simulink model "FullVehicleModel_ABS_ESP"  (R2019a)
settings: Solver=ode23s  StartTime=0.0  StopTime=t_f  MaxStep=0.1  RelTol=1e-3
values from neighbouring files (symbols this model uses):
  acc_US_test = 0    [mainVehicleModel.m]
  auxiliary_data = block.DialogPrm(3).Data    [FullVehicleModel_V3_sfun.m]    (also in mainVehicleModel.m = getAuxiliaryDataStruct())
  curv_akermann = 0    [mainVehicleModel.m]
  hv = 0.5    [mainVehicleModel.m]
  init_conditions_data = getInitialConditionsDataStruct( V_init )    [mainVehicleModel.m]
  lambda1_th = 0.2    [mainVehicleModel.m]
  lambda2_th = 0.1    [mainVehicleModel.m]
  maneuver_flag = 4    [mainVehicleModel.m]
  parametri_ABS = para    [ABSParameters.m]    (also in mainVehicleModel.m = ABSParameters(getVehicleDataStruct()))
  rho_off = 0.9    [mainVehicleModel.m]
  rho_on = 1.02    [mainVehicleModel.m]
  t_brake = t_f+1    (= 61)    [mainVehicleModel.m]
  Tb_dot_max = 5000    [mainVehicleModel.m]
  V_init = 50    [mainVehicleModel.m]
  v_on = 2.5    [mainVehicleModel.m]
  v_stop = 0.1    [mainVehicleModel.m]
  vehicle_data = block.DialogPrm(1).Data    [FullVehicleModel_V3_sfun.m]    (also in mainVehicleModel.m = getVehicleDataStruct())
undefined symbols (not defined in the file or in its folder): magnitude, sigbuilder_block
libraries: simulink x6, dspsigops x4
(part 1 of 2)
settings Model: Creator=luca  LastModifiedBy=LorenzoZappata
settings DataIOCC: SaveFormat=Array  ReturnWorkspaceOutputs=off
settings DebuggingCC: ArithmeticOperatorsInVariantConditions=warning
settings SFSimCC: SimUseLocalCustomCode=off
settings RTWCC: RTWUseLocalCustomCode=off
settings CodeAppCC: StateflowObjectComments=on

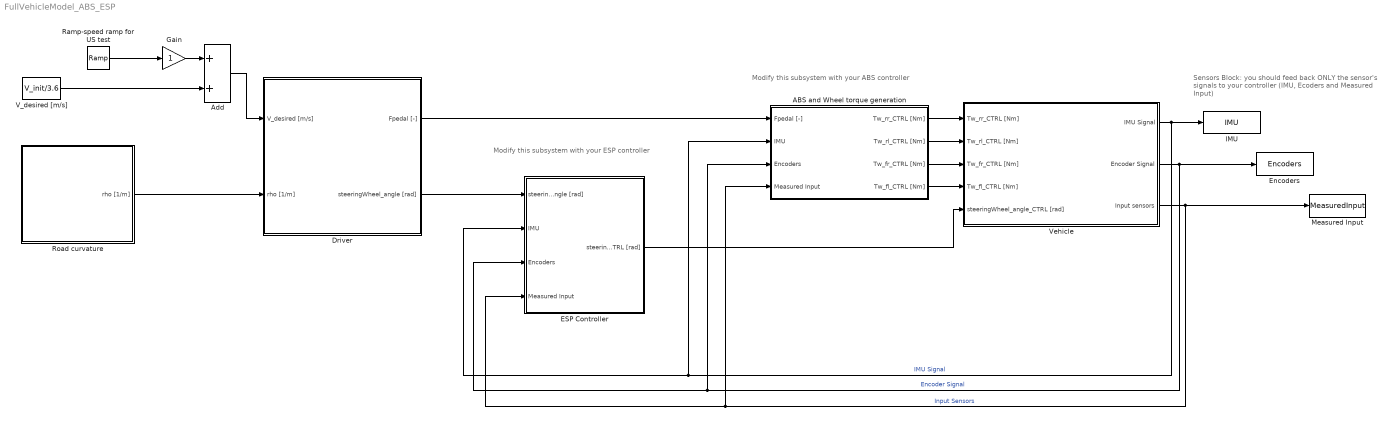
== system FullVehicleModel_ABS_ESP ==
  note: Modify this subsystem with your ABS controller
  note: Modify this subsystem with your ESP
      | controller
  note: Sensors Block: you should feed back ONLY
      | the sensor's signals to your controller
      | (IMU, Ecoders and Measured Input)
  ABS and Wheel torque generation : Subsystem
  Add : Sum
  Driver : Subsystem
  ESP Controller : Subsystem
  Encoders : ToWorkspace  VariableName=Encoders  SaveFormat=Timeseries  SampleTime=-1
  Gain : Gain
  IMU : ToWorkspace  VariableName=IMU  SaveFormat=Timeseries  SampleTime=-1
  Measured Input : ToWorkspace  VariableName=MeasuredInput  SaveFormat=Timeseries  SampleTime=-1
  Ramp-speed ramp for US test : simulink/Sources/Ramp  slope=acc_US_test  start=Tstart_US_test  InitialOutput=0
  Road curvature : Subsystem
  V_desired [m/s] : Constant  Value=V_init/3.6
  Vehicle : Subsystem
  wires:
  Driver/1(Fpedal [-]) -> ABS and Wheel torque generation/1(Fpedal [-])
  Driver/2(steeringWheel_angle [rad]) -> ESP Controller/1(steeringWheel_angle [rad])
  Vehicle/1(IMU Signal) -> IMU/1, ABS and Wheel torque generation/2(IMU), ESP Controller/2(IMU)  "IMU Signal"
  Vehicle/2(Encoder Signal) -> Encoders/1, ABS and Wheel torque generation/3(Encoders), ESP Controller/3(Encoders)  "Encoder Signal"
  Vehicle/3(Input sensors) -> Measured Input/1, ABS and Wheel torque generation/4(Measured Input), ESP Controller/4(Measured Input)  "Input Sensors"
  ESP Controller/1(steeringWheel_angle_CTRL [rad]) -> Vehicle/5(steeringWheel_angle_CTRL [rad])
  ABS and Wheel torque generation/4(Tw_fl_CTRL [Nm]) -> Vehicle/4(Tw_fl_CTRL [Nm])
  ABS and Wheel torque generation/3(Tw_fr_CTRL [Nm]) -> Vehicle/3(Tw_fr_CTRL [Nm])
  ABS and Wheel torque generation/2(Tw_rl_CTRL [Nm]) -> Vehicle/2(Tw_rl_CTRL [Nm])
  ABS and Wheel torque generation/1(Tw_rr_CTRL [Nm]) -> Vehicle/1(Tw_rr_CTRL [Nm])
  Ramp-speed ramp for US test/1 -> Gain/1
  V_desired [m/s]/1 -> Add/2
  Add/1 -> Driver/1(V_desired [m/s])
  Gain/1 -> Add/1
  Road curvature/1(rho [1/m]) -> Driver/2(rho [1/m])

== system FullVehicleModel_ABS_ESP/ABS and Wheel torque generation ==
  note: Insert your ABS design in the
      | following Subsystems
  Fpedal [-] : Inport
  IMU : Inport  Port=2
  Encoders : Inport  Port=3
  Measured Input : Inport  Port=4
  ABS Front Left Wheel : Subsystem
  ABS Front Right Wheel : Subsystem
  ABS Rear Left Wheel : Subsystem
  ABS Rear Right Wheel : Subsystem
  Accelerator : Subsystem
  Brake : Subsystem
  Demux : Demux
  Scope6 : Scope
  Switch : Switch
  Tw_rr_CTRL [Nm] : Outport
  Tw_rl_CTRL [Nm] : Outport  Port=2
  Tw_fr_CTRL [Nm] : Outport  Port=3
  Tw_fl_CTRL [Nm] : Outport  Port=4
  wires:
  Demux/2 -> ABS Rear Left Wheel/1(Tw_rl [Nm])
  Switch/1 -> Demux/1
  Demux/1 -> Scope6/1, ABS Rear Right Wheel/1(Tw_rr [Nm])
  Fpedal [-]/1 -> Brake/1(Fpedal [-]), Accelerator/1(Fpedal [-]), Switch/2
  ABS Rear Right Wheel/1(Tw_rr_CTRL [Nm]) -> Tw_rr_CTRL [Nm]/1
  Measured Input/1 -> ABS Front Left Wheel/4(Measured Input), ABS Front Right Wheel/4(Measured Input), ABS Rear Left Wheel/4(Measured Input), ABS Rear Right Wheel/4(Measured Input)
  Encoders/1 -> ABS Rear Right Wheel/3(Encoders), ABS Front Right Wheel/3(Encoders), ABS Front Left Wheel/3(Encoders), ABS Rear Left Wheel/3(Encoders)
  IMU/1 -> ABS Rear Left Wheel/2(IMU), ABS Front Left Wheel/2(IMU), ABS Front Right Wheel/2(IMU), ABS Rear Right Wheel/2(IMU)
  ABS Rear Left Wheel/1(Tw_rl_CTRL [Nm]) -> Tw_rl_CTRL [Nm]/1
  Demux/3 -> ABS Front Right Wheel/1(Tw_fr [Nm])
  ABS Front Right Wheel/1(Tw_rr_CTRL [Nm]) -> Tw_fr_CTRL [Nm]/1
  Demux/4 -> ABS Front Left Wheel/1(Tw_fl [Nm])
  ABS Front Left Wheel/1(Tw_rr_CTRL [Nm]) -> Tw_fl_CTRL [Nm]/1
  Accelerator/1(Tw [Nm]) -> Switch/1
  Brake/1(Tw [Nm]) -> Switch/3

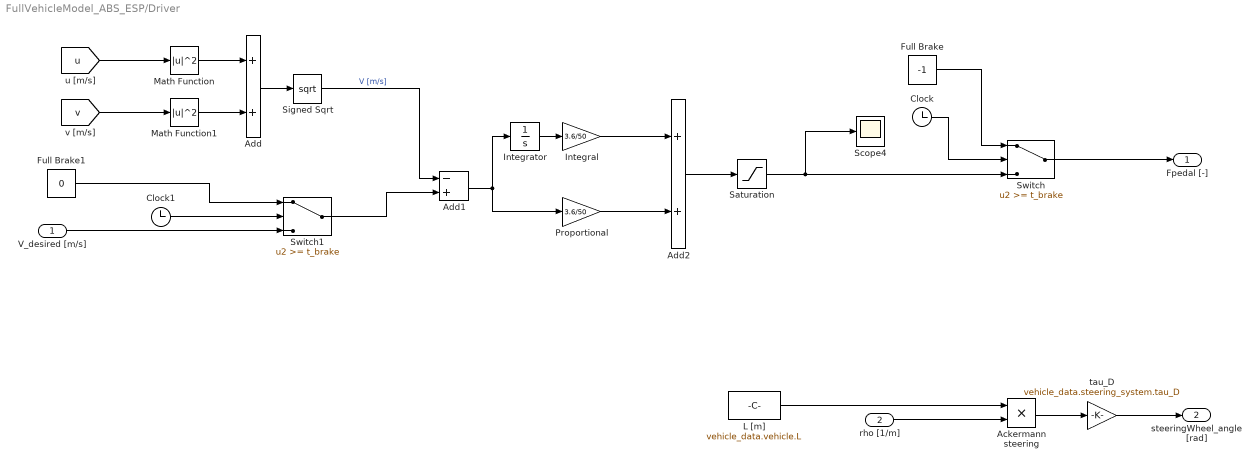
== system FullVehicleModel_ABS_ESP/Driver ==
  V_desired [m/s] : Inport
  rho [1/m] : Inport  Port=2
  Ackermann steering : Product  Inputs=**
  Add : Sum
  Add1 : Sum  Inputs=-+
  Add2 : Sum
  Clock : Clock
  Clock1 : Clock
  Full Brake : Constant  Value=-1
  Full Brake1 : Constant  Value=0
  Integral : Gain  Gain=3.6/50
  Integrator : Integrator
  L [m] : Constant  Value=vehicle_data.vehicle.L
  Math Function : Math  Operator=magnitude^2  SaturateOnIntegerOverflow=on
  Math Function1 : Math  Operator=magnitude^2  SaturateOnIntegerOverflow=on
  Proportional : Gain  Gain=3.6/50
  Saturation : Saturate  UpperLimit=1  LowerLimit=-1
  Scope4 : Scope
  Signed Sqrt : Sqrt  SaturateOnIntegerOverflow=on
  Switch : Switch  Threshold=t_brake
  Switch1 : Switch  Threshold=t_brake
  tau_D : Gain  Gain=vehicle_data.steering_system.tau_D
  Fpedal [-] : Outport
  steeringWheel_angle [rad] : Outport  Port=2
  wires:
  Proportional/1 -> Add2/2
  Add2/1 -> Saturation/1
  Integrator/1 -> Integral/1
  L [m]/1 -> Ackermann steering/1
  Add/1 -> Signed Sqrt/1
  Math Function1/1 -> Add/2
  Add1/1 -> Integrator/1, Proportional/1
  Signed Sqrt/1 -> Add1/1  "V [m/s]"
  Ackermann steering/1 -> tau_D/1
  Math Function/1 -> Add/1
  rho [1/m]/1 -> Ackermann steering/2
  Integral/1 -> Add2/1
  [u] -> Math Function/1
  [v] -> Math Function1/1
  V_desired [m/s]/1 -> Switch1/3
  Saturation/1 -> Switch/3, Scope4/1
  Full Brake1/1 -> Switch1/1
  Clock1/1 -> Switch1/2
  Full Brake/1 -> Switch/1
  Clock/1 -> Switch/2
  Switch/1 -> Fpedal [-]/1
  Switch1/1 -> Add1/2
  tau_D/1 -> steeringWheel_angle [rad]/1

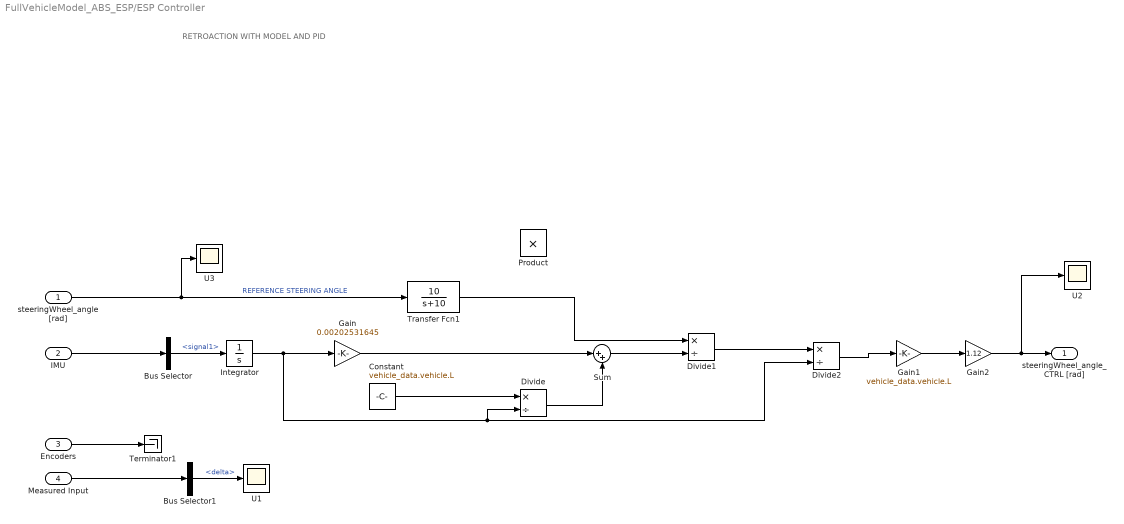
== system FullVehicleModel_ABS_ESP/ESP Controller ==
  note: RETROACTION WITH MODEL AND PID
  steeringWheel_angle [rad] : Inport
  IMU : Inport  Port=2
  Encoders : Inport  Port=3
  Measured Input : Inport  Port=4
  Bus Selector : BusSelector  OutputSignals=signal1
  Bus Selector1 : BusSelector  OutputSignals=delta
  Constant : Constant  Value=vehicle_data.vehicle.L
  Divide : Product  Inputs=*/
  Divide1 : Product  Inputs=*/
  Divide2 : Product  Inputs=*/
  Gain : Gain  Gain=0.00202531645
  Gain1 : Gain  Gain=vehicle_data.vehicle.L
  Gain2 : Gain  Gain=1.12
  Integrator : Integrator  InitialCondition=V_init/3.6
  Product : Product
  Sum : Sum  Inputs=|++
  Terminator1 : Terminator
  Transfer Fcn1 : TransferFcn  Numerator=[10]  Denominator=[1 10]
  U1 : Scope
  U2 : Scope
  U3 : Scope
  steeringWheel_angle_CTRL [rad] : Outport
  wires:
  Encoders/1 -> Terminator1/1
  Measured Input/1 -> Bus Selector1/1
  Integrator/1 -> Gain/1, Divide2/2, Divide/2
  IMU/1 -> Bus Selector/1
  Bus Selector/1 -> Integrator/1  "<signal1>"
  steeringWheel_angle [rad]/1 -> Transfer Fcn1/1, U3/1  "REFERENCE STEERING ANGLE"
  Constant/1 -> Divide/1
  Gain/1 -> Sum/1
  Divide/1 -> Sum/2
  Sum/1 -> Divide1/2
  Divide1/1 -> Divide2/1
  Divide2/1 -> Gain1/1
  Gain2/1 -> U2/1, steeringWheel_angle_CTRL [rad]/1
  Gain1/1 -> Gain2/1
  Transfer Fcn1/1 -> Divide1/1
  Bus Selector1/1 -> U1/1  "<delta>"

== system FullVehicleModel_ABS_ESP/Road curvature ==
  1/(tau_D) : Gain  Gain=1/(vehicle_data.steering_system.tau_D)
  1/(tau_D)1 : Gain  Gain=1/(vehicle_data.steering_system.tau_D)
  1/(tau_D)2 : Gain  Gain=1/(vehicle_data.steering_system.tau_D)
  Brake Maneuver : Constant  Value=0
  Constant curvature Maneuver : Subsystem  Tag=STV Subsys  LoadFcn=sigbuilder_block('load');  StartFcn=sigbuilder_block('start');  StopFcn=sigbuilder_block('stop');  ClipboardFcn=sigbuilder_block('clipboard');  mask(Sigbuilder block){tuvar=[0:10]}
      mask help: Simulink:masks:SigbuilderBlock_MD
      mask init:
      | if ~strcmp(get_param(bdroot(gcbh),'SimulationStatus'),'stopped') tuvar = sigbuilder_block('maskInit'); end
      settings: CopyFcn=sigbuilder_block('copy');  DeleteFcn=sigbuilder_block('delete');  ModelCloseFcn=sigbuilder_block('modelClose');  PreSaveFcn=sigbuilder_block('preSave');  PauseFcn=sigbuilder_block('pause');  ContinueFcn=sigbuilder_block('continue');  NameChangeFcn=sigbuilder_block('namechange');  OpenFcn=sigbuilder_block('open',[0 0 1319 754 ]);  CloseFcn=sigbuilder_block('close');
      mask Display: plot(0, 0, 100, 100,[2, 2, 32, 32, 2], [68, 8, 8, 68, 68],[32, 2], [38, 38], [32, 19, 2],[53, 60, 44], [32, 17, 17, 2],[16, 16, 31, 31]);txt = getActiveGroup(gcbh);text(2, 100, txt,'verticalAlignment', 'top');
  Desired curvature  [1/m] : Constant  Value=curv_akermann
  Double Lane Change Maneuver : Subsystem  Tag=STV Subsys  LoadFcn=sigbuilder_block('load');  StartFcn=sigbuilder_block('start');  StopFcn=sigbuilder_block('stop');  ClipboardFcn=sigbuilder_block('clipboard');  mask(Sigbuilder block){tuvar=[0:10]}
      mask help: Simulink:masks:SigbuilderBlock_MD
      mask init:
      | if ~strcmp(get_param(bdroot(gcbh),'SimulationStatus'),'stopped') tuvar = sigbuilder_block('maskInit'); end
      settings: CopyFcn=sigbuilder_block('copy');  DeleteFcn=sigbuilder_block('delete');  ModelCloseFcn=sigbuilder_block('modelClose');  PreSaveFcn=sigbuilder_block('preSave');  PauseFcn=sigbuilder_block('pause');  ContinueFcn=sigbuilder_block('continue');  NameChangeFcn=sigbuilder_block('namechange');  OpenFcn=sigbuilder_block('open',[0 0 1280 649 ]);  CloseFcn=sigbuilder_block('close');
      mask Display: plot(0, 0, 100, 100,[2, 2, 32, 32, 2], [68, 8, 8, 68, 68],[32, 2], [38, 38], [32, 19, 2],[53, 60, 44], [32, 17, 17, 2],[16, 16, 31, 31]);txt = getActiveGroup(gcbh);text(2, 100, txt,'verticalAlignment', 'top');
  Maneuver Flag : Constant  Value=maneuver_flag
  Multiport Switch : MultiPortSwitch  Inputs=4
  Product : Product
  Step : Step  SampleTime=0
  rho [1/m] : Outport
  wires:
  Brake Maneuver/1 -> 1/(tau_D)/1
  Maneuver Flag/1 -> Multiport Switch/1
  Constant curvature Maneuver/1(Signal 1) -> 1/(tau_D)2/1
  Double Lane Change Maneuver/1(Signal 1) -> 1/(tau_D)1/1
  Multiport Switch/1 -> rho [1/m]/1
  Desired curvature  [1/m]/1 -> Product/2
  Product/1 -> Multiport Switch/5
  Step/1 -> Product/1
  1/(tau_D)/1 -> Multiport Switch/2
  1/(tau_D)1/1 -> Multiport Switch/3
  1/(tau_D)2/1 -> Multiport Switch/4

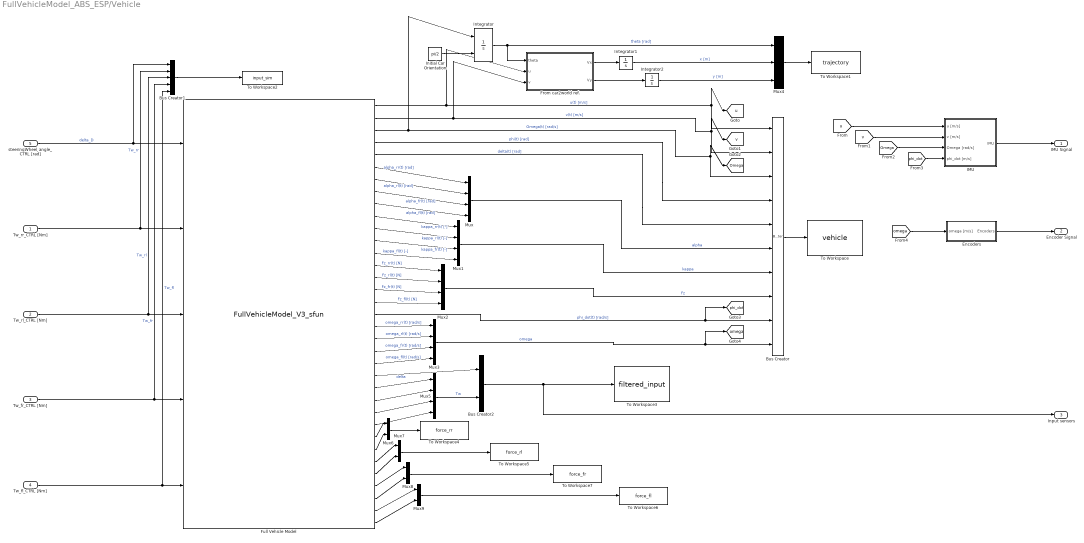
== system FullVehicleModel_ABS_ESP/Vehicle ==
  Tw_rr_CTRL [Nm] : Inport
  Tw_rl_CTRL [Nm] : Inport  Port=2
  Tw_fr_CTRL [Nm] : Inport  Port=3
  Tw_fl_CTRL [Nm] : Inport  Port=4
  steeringWheel_angle_CTRL [rad] : Inport  Port=5
  Bus Creator : BusCreator  Inputs=10
  Bus Creator1 : BusCreator  Inputs=5
  Bus Creator2 : BusCreator  Inputs=2
  Encoders : Subsystem
  "From car2world ref. " : Subsystem
  Full Vehicle Model : M-S-Function  FunctionName=FullVehicleModel_V3_sfun  Parameters=vehicle_data, init_conditions_data, auxiliary_data  mask(Matlab S-function:FullVehicleModel_V3_sfun){vehicle_data=vehicle_data, init_conditions_data=init_conditions_data, auxiliary_data=auxiliary_data}
      mask prompts: vehicle_data "Vehicle data structure"; init_conditions_data "Initial conditions structure"; auxiliary_data "Auxiliary data"
      mask help: This is a level-2 MATLAB file S-function that implements full vehicle dynamics at high and low speeds. This includes the vertical and lateral dynamics, together with wheel dynamics (wheels speed, lateral and longitudinal slip) and roll dynamics.
      mask Display:
      | port_label('input', 1, 'delta_D [rad]');
      | port_label('input', 2, 'Tw_rr [Nm]');
      | port_label('input', 3, 'Tw_rl [Nm]');
      | port_label('input', 4, 'Tw_fr [Nm]');
      | port_label('input', 5, 'Tw_fl [Nm]');
      | 
      | % x(1)  = u(t)        -> Longitudinal vehicle velocity
      | port_label('output', 1, 'u [m/s]');
      | % x(2)  = v(t)        -> Lateral vehicle velocity
      | port_label('output', 2, 'v [m/s]');
      | % x(3)  = Omega(t)    -> Yaw rate
      | port_label('output', 3, 'Omega [rad/s]');
      | % x(4)  = phi(t)      -> Roll angle
      | port_label('output', 4, 'phi [rad]');
      | % x(5)  = delta(t)    -> Steering angle
      | port_label('output', 5, 'delta [rad]');
      | % x(6)  = alpha_rr(t) -> Side slip angle, rear right wheel
      | port_label('output', 6, 'alpha_rr [-]');
      | % x(7)  = alpha_rl(t) -> Side slip angle, rear left wheel
      | port_label('output', 7, 'alpha_rl [-]');
      | % x(8)  = alpha_fr(t) -> Side slip angle, front right wheel
      | port_label('output', 8, 'alpha_fr [-]');
      | % x(9)  = alpha_fl(t) -> Side slip angle, front left wheel
      | port_label('output', 9, 'alpha_fl [-]');
      | % x(10) = kappa_rr(t) -> Longitudinal slip, rear right wheel
      | port_label('output', 10, 'kappa_rr [-]');
      | % x(11) = kappa_rl(t) -> Longitudinal slip, rear left wheel
      | port_label('output', 11, 'kappa_rl [-]');
      | % x(12) = kappa_fr(t) -> Longitudinal slip, front right wheel
      | port_label('output', 12, 'kappa_fr [-]');
      | % x(13) = kappa_fl(t) -> Longitudinal slip, front left wheel
      | port_label('output', 13, 'kappa_fl [-]');
      | % x(14) = Fz_rr(t)    -> Vertical load, rear right wheel
      | port_label('output', 14, 'Fz_rr [N]');
      | % x(15) = Fz_rl(t)    -> Vertical load, rear rear left wheel
      | port_label('output', 15, 'Fz_rl [N]');
      | % x(16) = Fz_fr(t)    -> Vertical load, front right wheel
      | port_label('output', 16, 'Fz_fr [N]');
      | % x(17) = Fz_fl(t)    -> Vertical load, front left wheel
      | port_label('output', 17, 'Fz_fl [N]');
      | % x(18) = phi_dot(t)  -> Roll rate
      | port_label('output', 18, 'phi_dot [rad/s]');
      | % x(19) = omega_rr(t) -> angular velocity rear right wheel
      | port_label('output', 19, 'omega_rr [rad/s]');
      | % x(20) = omega_rl(t) -> angular velocity rear left wheel
      | port_label('output', 20, 'omega_rl [rad/s]');
      | % x(21) = omega_fr(t) -> angular velocity front right wheel
      | port_label('output', 21, 'omega_fr [rad/s]');
      | % x(22) = omega_fl(t) -> angular velocity front left wheel
      | port_label('output', 22, 'omega_fl [rad/s]');
      | % x(23) = delta(t) -> real steer angle
      | port_label('output', 23, 'delta [rad]');
      | % x(24:27) = Tw(t) -> Filtered wheel torque
      | port_label('output', 24, 'Tw_rr [Nm]');
      | port_label('output', 25, 'Tw_rl [Nm]');
      | port_label('output', 26, 'Tw_fr [Nm]');
      | port_label('output', 27, 'Tw_fl [Nm]');
      | 
      | % Wheel forces
      | % Rear Right
      | port_label('output', 28, 'Fx_rr [N]');
      | port_label('output', 29, 'Fy_rr [N]');
      | % Rear Left
      | port_label('output', 30, 'Fx_rl [N]');
      | port_label('output', 31, 'Fy_rl [N]');
      | % Front Right
      | port_label('output', 32, 'Fx_fr [N]');
      | port_label('output', 33, 'Fy_fr [N]');
      | % Front Left
      | port_label('output', 34, 'Fx_fl [N]');
      | port_label('output', 35, 'Fy_fl [N]');
  IMU : Subsystem
  Initial Car Orientation : Constant  Value=pi/2
  Integrator : Integrator  InitialConditionSource=external
  Integrator1 : Integrator
  Integrator2 : Integrator
  Mux{,1..3,5} (5 alike) : Mux
  Mux4 : Mux  Inputs=3
  Mux{6..9} (4 alike) : Mux  Inputs=2
  To Workspace : ToWorkspace  VariableName=vehicle  SaveFormat=Timeseries  SampleTime=-1
  To Workspace1 : ToWorkspace  VariableName=trajectory  SaveFormat=Timeseries  SampleTime=-1
  To Workspace2 : ToWorkspace  VariableName=input_sim  SaveFormat=Timeseries  SampleTime=-1
  To Workspace3 : ToWorkspace  VariableName=filtered_input  SaveFormat=Timeseries  SampleTime=-1
  To Workspace4 : ToWorkspace  VariableName=force_rr  SaveFormat=Timeseries  SampleTime=-1
  To Workspace5 : ToWorkspace  VariableName=force_rl  SaveFormat=Timeseries  SampleTime=-1
  To Workspace6 : ToWorkspace  VariableName=force_fl  SaveFormat=Timeseries  SampleTime=-1
  To Workspace7 : ToWorkspace  VariableName=force_fr  SaveFormat=Timeseries  SampleTime=-1
  IMU Signal : Outport
  Encoder Signal : Outport  Port=2
  Input sensors : Outport  Port=3
  tag scope: Omega=global, omega=global, phi_dot=global, u=global, v=global
  wires:
  Mux5/1 -> Bus Creator2/2  "Tw"
  Full Vehicle Model/4 -> Bus Creator/4  "phi(t) [rad]"
  Integrator/1 -> "From car2world ref. "/1(theta), Mux4/1  "theta [rad]"
  Mux8/1 -> To Workspace7/1
  Full Vehicle Model/32 -> Mux8/1
  Mux2/1 -> Bus Creator/8  "Fz"
  "From car2world ref. "/1(Vx) -> Integrator1/1
  Full Vehicle Model/28 -> Mux6/1
  Full Vehicle Model/35 -> Mux9/2
  Full Vehicle Model/19 -> Mux3/1  "omega_rr(t) [rad/s]"
  Mux7/1 -> To Workspace5/1
  Mux9/1 -> To Workspace6/1
  Bus Creator/1 -> To Workspace/1
  Full Vehicle Model/6 -> Mux/1  "alpha_rr(t) [rad]"
  Full Vehicle Model/2 -> [v], Bus Creator/2, "From car2world ref. "/3(v)  "v(t) [m/s]"
  Full Vehicle Model/7 -> Mux/2  "alpha_rl(t) [rad]"
  Full Vehicle Model/12 -> Mux1/3  "kappa_fr(t) [-]"
  Full Vehicle Model/20 -> Mux3/2  "omega_rl(t) [rad/s]"
  Full Vehicle Model/16 -> Mux2/3  "Fz_fr(t) [N]"
  Full Vehicle Model/9 -> Mux/4  "alpha_fl(t) [rad]"
  Full Vehicle Model/10 -> Mux1/1  "kappa_rr(t) [-]"
  Full Vehicle Model/11 -> Mux1/2  "kappa_rl(t) [-]"
  Full Vehicle Model/31 -> Mux7/2
  Full Vehicle Model/26 -> Mux5/3
  Full Vehicle Model/24 -> Mux5/1
  Full Vehicle Model/23 -> Bus Creator2/1  "delta"
  Full Vehicle Model/8 -> Mux/3  "alpha_fr(t) [rad]"
  Initial Car Orientation/1 -> Integrator/2
  Full Vehicle Model/22 -> Mux3/4  "omega_fl(t) [rad/s]"
  Bus Creator2/1 -> Input sensors/1, To Workspace3/1
  Full Vehicle Model/29 -> Mux6/2
  Full Vehicle Model/5 -> Bus Creator/5  "delta(t) [rad]"
  Full Vehicle Model/21 -> Mux3/3  "omega_fr(t) [rad/s]"
  Full Vehicle Model/3 -> [Omega], Bus Creator/3, Integrator/1  "Omega(t) [rad/s]"
  Mux3/1 -> Bus Creator/10, [omega]  "omega"
  Full Vehicle Model/1 -> [u], Bus Creator/1, "From car2world ref. "/2(u)  "u(t) [m/s]"
  Full Vehicle Model/13 -> Mux1/4  "kappa_fl(t) [-]"
  Mux4/1 -> To Workspace1/1
  Bus Creator1/1 -> To Workspace2/1
  steeringWheel_angle_CTRL [rad]/1 -> Bus Creator1/1, Full Vehicle Model/1  "delta_D"
  Full Vehicle Model/18 -> Bus Creator/9, [phi_dot]  "phi_dot(t) [rad/s]"
  Full Vehicle Model/30 -> Mux7/1
  Integrator2/1 -> Mux4/3  "y [m]"
  Mux6/1 -> To Workspace4/1
  Mux/1 -> Bus Creator/6  "alpha"
  Full Vehicle Model/27 -> Mux5/4
  Full Vehicle Model/17 -> Mux2/4  "Fz_fl(t) [N]"
  Integrator1/1 -> Mux4/2  "x [m]"
  "From car2world ref. "/2(Vy) -> Integrator2/1
  Full Vehicle Model/14 -> Mux2/1  "Fz_rr(t) [N]"
  Mux1/1 -> Bus Creator/7  "kappa"
  Full Vehicle Model/25 -> Mux5/2
  Full Vehicle Model/15 -> Mux2/2  "Fz_rl(t) [N]"
  Full Vehicle Model/34 -> Mux9/1
  Full Vehicle Model/33 -> Mux8/2
  Tw_rr_CTRL [Nm]/1 -> Bus Creator1/2, Full Vehicle Model/2  "Tw_rr"
  Tw_rl_CTRL [Nm]/1 -> Bus Creator1/3, Full Vehicle Model/3  "Tw_rl"
  Tw_fr_CTRL [Nm]/1 -> Bus Creator1/4, Full Vehicle Model/4  "Tw_fr"
  Tw_fl_CTRL [Nm]/1 -> Bus Creator1/5, Full Vehicle Model/5  "Tw_fl"
  [u] -> IMU/1(u [m/s])
  [v] -> IMU/2(v [m/s])
  IMU/1(IMU) -> IMU Signal/1
  [Omega] -> IMU/3(Omega [rad/s])
  [phi_dot] -> IMU/4(phi_dot [m/s])
  [omega] -> Encoders/1(omega [m/s])
  Encoders/1(Encoders) -> Encoder Signal/1

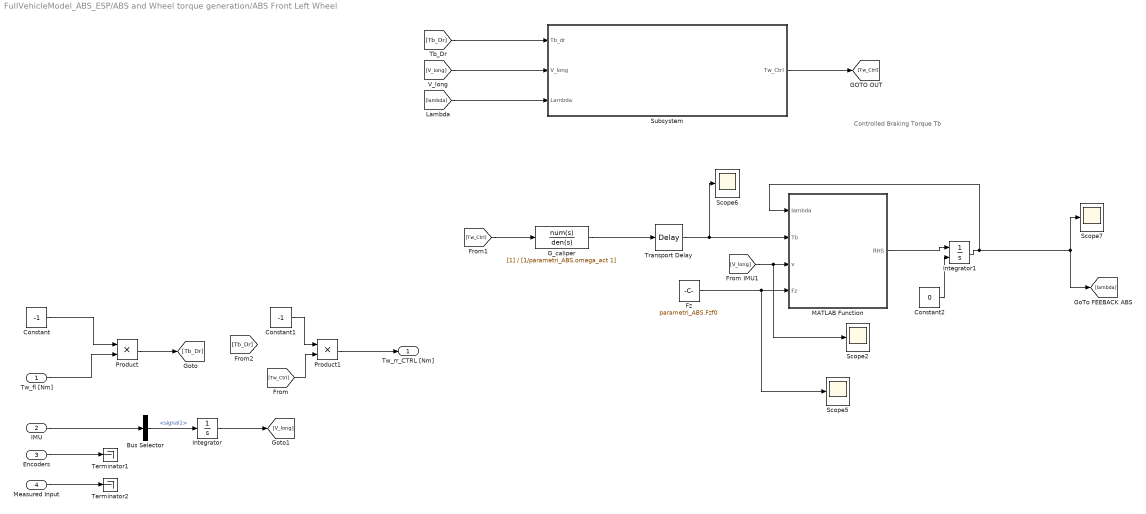
== system FullVehicleModel_ABS_ESP/ABS and Wheel torque generation/ABS Front Left Wheel ==
  note: Controlled Braking Torque Tb
  Tw_fl [Nm] : Inport
  IMU : Inport  Port=2
  Encoders : Inport  Port=3
  Measured Input : Inport  Port=4
  Bus Selector : BusSelector  OutputSignals=signal1
  Constant : Constant  Value=-1
  Constant1 : Constant  Value=-1
  Constant2 : Constant  Value=0
  Fz : Constant  Value=parametri_ABS.Fzf0
  G_caliper : TransferFcn  Denominator=[1/parametri_ABS.omega_act 1]
  Integrator : Integrator  InitialCondition=V_init
  Integrator1 : Integrator  InitialConditionSource=external
  MATLAB Function : MATLAB Function  TreatAsAtomicUnit=on
  Product : Product
  Product1 : Product
  Scope{2,5..7} (4 alike) : Scope
  Subsystem : Subsystem
  Terminator1 : Terminator
  Terminator2 : Terminator
  Transport Delay : TransportDelay  DelayTime=parametri_ABS.tau_delay  BufferSize=10000
  Tw_rr_CTRL [Nm] : Outport
  wires:
  Encoders/1 -> Terminator1/1
  Measured Input/1 -> Terminator2/1
  IMU/1 -> Bus Selector/1
  Constant/1 -> Product/1
  Tw_fl [Nm]/1 -> Product/2
  Fz/1 -> Scope5/1, MATLAB Function/4(Fz)
  MATLAB Function/1(RHS) -> Integrator1/1
  [V_long] -> Scope2/1, MATLAB Function/3(v)
  G_caliper/1 -> Transport Delay/1
  Integrator1/1 -> [lambda], Scope7/1, MATLAB Function/1(lambda)
  [Tb_Dr] -> Subsystem/1(Tb_dr)
  Transport Delay/1 -> Scope6/1, MATLAB Function/2(Tb)
  [Tw_Ctrl] -> G_caliper/1
  [lambda] -> Subsystem/3(Lambda)
  Subsystem/1(Tw_Ctrl) -> [Tw_Ctrl]
  [V_long] -> Subsystem/2("V_long ")
  Constant2/1 -> Integrator1/2
  Product/1 -> [Tb_Dr]
  Constant1/1 -> Product1/1
  Product1/1 -> Tw_rr_CTRL [Nm]/1
  Bus Selector/1 -> Integrator/1  "<signal1>"
  Integrator/1 -> [V_long]
  [Tw_Ctrl] -> Product1/2

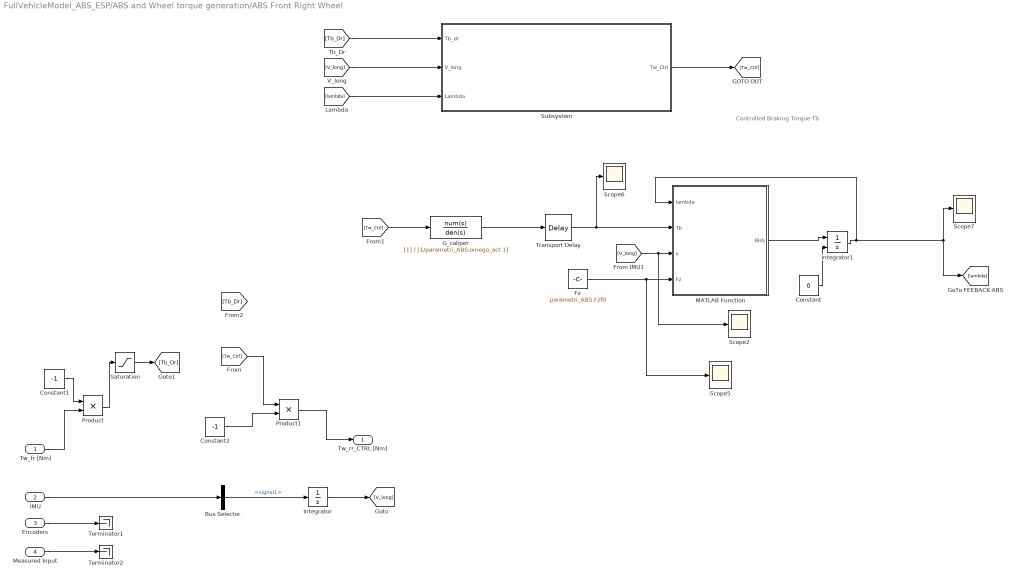
== system FullVehicleModel_ABS_ESP/ABS and Wheel torque generation/ABS Front Right Wheel ==
  note: Controlled Braking Torque Tb
  Tw_fr [Nm] : Inport
  IMU : Inport  Port=2
  Encoders : Inport  Port=3
  Measured Input : Inport  Port=4
  Bus Selector : BusSelector  OutputSignals=signal1
  Constant : Constant  Value=0
  Constant1 : Constant  Value=-1
  Constant2 : Constant  Value=-1
  Fz : Constant  Value=parametri_ABS.Fzf0
  G_caliper : TransferFcn  Denominator=[1/parametri_ABS.omega_act 1]
  Integrator : Integrator  InitialCondition=V_init/3.6
  Integrator1 : Integrator  InitialConditionSource=external
  MATLAB Function : MATLAB Function  TreatAsAtomicUnit=on
  Product : Product
  Product1 : Product
  Saturation : Saturate  UpperLimit=1500  LowerLimit=0
  Scope{2,5..7} (4 alike) : Scope
  Subsystem : Subsystem
  Terminator1 : Terminator
  Terminator2 : Terminator
  Transport Delay : TransportDelay  DelayTime=parametri_ABS.tau_delay  BufferSize=10000
  Tw_rr_CTRL [Nm] : Outport
  wires:
  IMU/1 -> Bus Selector/1
  Measured Input/1 -> Terminator2/1
  Encoders/1 -> Terminator1/1
  [V_long] -> Scope2/1, MATLAB Function/3(v)
  MATLAB Function/1(RHS) -> Integrator1/1
  [lambda] -> Subsystem/3(Lambda)
  Constant/1 -> Integrator1/2
  [Tw_Ctrl] -> G_caliper/1
  Transport Delay/1 -> Scope6/1, MATLAB Function/2(Tb)
  G_caliper/1 -> Transport Delay/1
  [V_long] -> Subsystem/2("V_long ")
  Fz/1 -> Scope5/1, MATLAB Function/4(Fz)
  [Tb_Dr] -> Subsystem/1(Tb_dr)
  Integrator1/1 -> [lambda], Scope7/1, MATLAB Function/1(lambda)
  Subsystem/1(Tw_Ctrl) -> [Tw_Ctrl]
  Bus Selector/1 -> Integrator/1  "<signal1>"
  Integrator/1 -> [V_long]
  Constant2/1 -> Product1/2
  Product1/1 -> Tw_rr_CTRL [Nm]/1
  Constant1/1 -> Product/1
  Product/1 -> Saturation/1
  Saturation/1 -> [Tb_Dr]
  Tw_fr [Nm]/1 -> Product/2
  [Tw_Ctrl] -> Product1/1

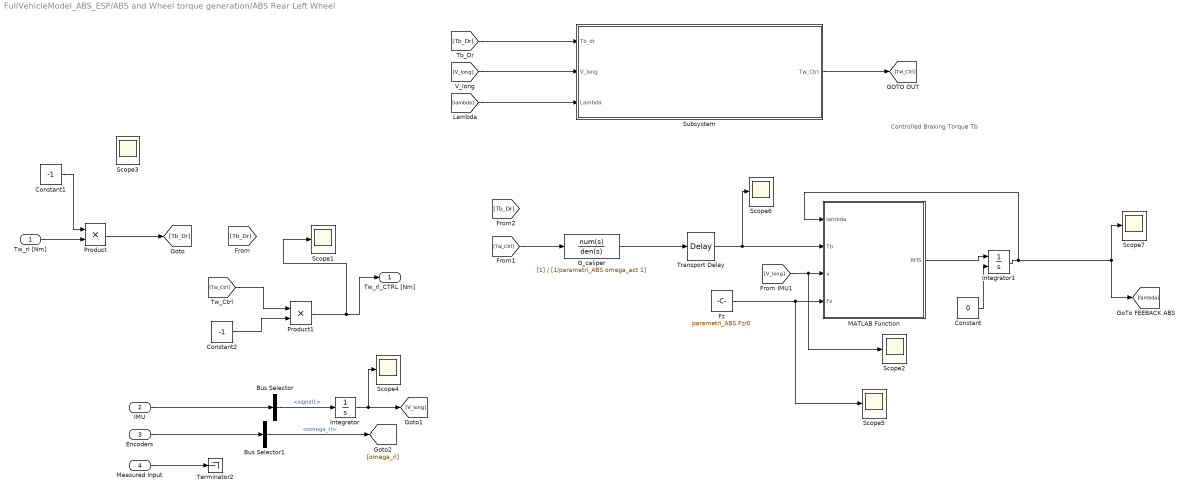
== system FullVehicleModel_ABS_ESP/ABS and Wheel torque generation/ABS Rear Left Wheel ==
  note: Controlled Braking Torque Tb
  Tw_rl [Nm] : Inport
  IMU : Inport  Port=2
  Encoders : Inport  Port=3
  Measured Input : Inport  Port=4
  Bus Selector : BusSelector  OutputSignals=signal1
  Bus Selector1 : BusSelector  OutputSignals=omega_rl
  Constant : Constant  Value=0
  Constant1 : Constant  Value=-1
  Constant2 : Constant  Value=-1
  Fz : Constant  Value=parametri_ABS.Fzr0
  G_caliper : TransferFcn  Denominator=[1/parametri_ABS.omega_act 1]
  Integrator : Integrator  InitialCondition=V_init/3.6
  Integrator1 : Integrator  InitialConditionSource=external
  MATLAB Function : MATLAB Function  TreatAsAtomicUnit=on
  Product : Product
  Product1 : Product
  Scope{1..7} (7 alike) : Scope
  Subsystem : Subsystem
  Terminator2 : Terminator
  Transport Delay : TransportDelay  DelayTime=parametri_ABS.tau_delay  BufferSize=10000
  Tw_rl_CTRL [Nm] : Outport
  wires:
  Encoders/1 -> Bus Selector1/1
  Measured Input/1 -> Terminator2/1
  IMU/1 -> Bus Selector/1
  Constant1/1 -> Product/1
  Tw_rl [Nm]/1 -> Product/2
  Bus Selector/1 -> Integrator/1  "<signal1>"
  Integrator/1 -> Scope4/1, [V_long]
  Bus Selector1/1 -> [omega_rl]  "<omega_rl>"
  Constant2/1 -> Product1/2
  [V_long] -> Scope2/1, MATLAB Function/3(v)
  MATLAB Function/1(RHS) -> Integrator1/1
  [lambda] -> Subsystem/3(Lambda)
  Constant/1 -> Integrator1/2
  Transport Delay/1 -> Scope6/1, MATLAB Function/2(Tb)
  G_caliper/1 -> Transport Delay/1
  [V_long] -> Subsystem/2("V_long ")
  Fz/1 -> Scope5/1, MATLAB Function/4(Fz)
  [Tb_Dr] -> Subsystem/1(Tb_dr)
  Integrator1/1 -> [lambda], Scope7/1, MATLAB Function/1(lambda)
  Subsystem/1(Tw_Ctrl) -> [Tw_Ctrl]
  Product/1 -> [Tb_Dr]
  Product1/1 -> Tw_rl_CTRL [Nm]/1, Scope1/1
  [Tw_Ctrl] -> G_caliper/1
  [Tw_Ctrl] -> Product1/1

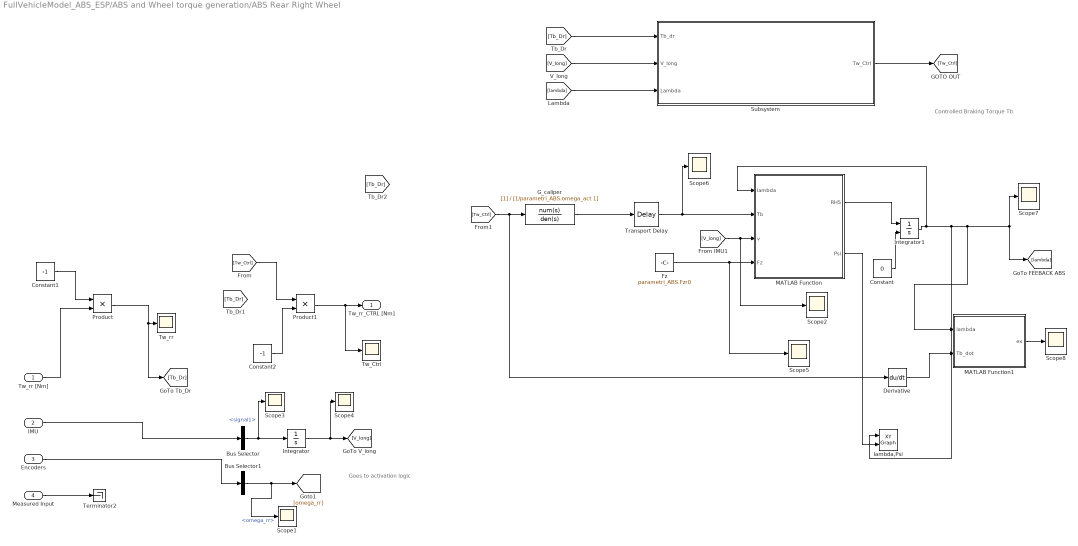
== system FullVehicleModel_ABS_ESP/ABS and Wheel torque generation/ABS Rear Right Wheel ==
  note: Goes to activation logic
  note: Controlled Braking Torque Tb
  Tw_rr [Nm] : Inport
  IMU : Inport  Port=2
  Encoders : Inport  Port=3
  Measured Input : Inport  Port=4
  Bus Selector : BusSelector  OutputSignals=signal1
  Bus Selector1 : BusSelector  OutputSignals=omega_rr
  Constant : Constant  Value=0
  Constant1 : Constant  Value=-1
  Constant2 : Constant  Value=-1
  Derivative : Derivative
  Fz : Constant  Value=parametri_ABS.Fzr0
  G_caliper : TransferFcn  Denominator=[1/parametri_ABS.omega_act 1]
  Integrator : Integrator  InitialCondition=V_init/3.6
  Integrator1 : Integrator  InitialConditionSource=external
  MATLAB Function : MATLAB Function  TreatAsAtomicUnit=on
  MATLAB Function1 : MATLAB Function  TreatAsAtomicUnit=on
  Product : Product
  Product1 : Product
  Scope{1..8} (8 alike) : Scope
  Subsystem : Subsystem
  Terminator2 : Terminator
  Transport Delay : TransportDelay  DelayTime=parametri_ABS.tau_delay  BufferSize=10000
  "Tw_Ctrl " : Scope
  Tw_rr : Scope
  lambda,Psi : simulink/Sinks/XY Graph  xmin=0  xmax=1  ymin=0  ymax=4000  st=-1
  Tw_rr_CTRL [Nm] : Outport
  wires:
  IMU/1 -> Bus Selector/1
  Measured Input/1 -> Terminator2/1
  Encoders/1 -> Bus Selector1/1
  Bus Selector/1 -> Scope3/1, Integrator/1  "<signal1>"
  Integrator/1 -> Scope4/1, [V_long]
  G_caliper/1 -> Transport Delay/1
  Bus Selector1/1 -> Scope1/1, [omega_rr]  "<omega_rr>"
  [V_long] -> Scope2/1, MATLAB Function/3(v)
  MATLAB Function/1(RHS) -> Integrator1/1
  Transport Delay/1 -> Scope6/1, MATLAB Function/2(Tb)
  Subsystem/1(Tw_Ctrl) -> [Tw_Ctrl]
  [Tb_Dr] -> Subsystem/1(Tb_dr)
  [V_long] -> Subsystem/2("V_long ")
  [lambda] -> Subsystem/3(Lambda)
  Constant/1 -> Integrator1/2
  Fz/1 -> Scope5/1, MATLAB Function/4(Fz)
  Constant1/1 -> Product/1
  Integrator1/1 -> lambda,Psi/1, MATLAB Function1/1(lambda), [lambda], Scope7/1, MATLAB Function/1(lambda)
  Constant2/1 -> Product1/2
  Tw_rr [Nm]/1 -> Product/2
  Product1/1 -> "Tw_Ctrl "/1, Tw_rr_CTRL [Nm]/1
  Product/1 -> [Tb_Dr], Tw_rr/1
  MATLAB Function1/1(ex) -> Scope8/1
  MATLAB Function/2(Psi) -> lambda,Psi/2
  Derivative/1 -> MATLAB Function1/2(Tb_dot)
  [Tw_Ctrl] -> Derivative/1, G_caliper/1
  [Tw_Ctrl] -> Product1/1

== system FullVehicleModel_ABS_ESP/ABS and Wheel torque generation/Accelerator ==
  Fpedal [-] : Inport
  1-D Lookup Table : Lookup_n-D  NumberOfTableDimensions=1  BreakpointsForDimension1=linspace(0,250/3.6,31)  Table=|  InternalRulePriority=Speed  RndMeth=Simplest  InputSameDT=on
      | 500*[0.442662657646371
      | 0.537281800718283
      | 0.631900943790195
      | 0.726520086862107
      | 0.821139229934018
      | 0.859929256634989
      | 0.897666213627126
      | 0.918905078514199
      | 0.939980602614386
      | 0.959177707665377
      | 0.977316148834879
      | 0.987691054873465
      | 0.996795820900055
      | 1
      | 0.995733117962017
      | 0.989286574404060
      | 0.982840030846103
      | 0.974205033220170
      | 0.965525373266320
      | 0.956088102993640
      | 0.944254781591915
      | 0.930421573540466
      | 0.913474919507860
      | 0.895654110637824
      | 0.877209833235892
      | 0.858765555833960
      | 0.840321278432028
      | 0.817183521078455
      | 0.778999480858075
      | 0.389499740429037
      | 0]
  Add : Sum
  Constant : Constant  Value=0
  Math Function : Math  Operator=magnitude^2  SaturateOnIntegerOverflow=on
  Math Function1 : Math  Operator=magnitude^2  SaturateOnIntegerOverflow=on
  Mux10 : Mux
  Product : Product
  Saturation1 : Saturate  UpperLimit=1  LowerLimit=0
  Scope3 : Scope
  Scope4 : Scope
  Scope5 : Scope
  Signed Sqrt : Sqrt  SaturateOnIntegerOverflow=on
  Tw [Nm] : Outport
  wires:
  1-D Lookup Table/1 -> Scope5/1, Product/1
  Fpedal [-]/1 -> Saturation1/1
  Constant/1 -> Mux10/4, Mux10/3  "Tw_f"
  [v] -> Math Function1/1
  Signed Sqrt/1 -> Scope4/1, 1-D Lookup Table/1  "V"
  [u] -> Math Function/1
  Math Function/1 -> Add/1
  Product/1 -> Mux10/2, Mux10/1  "Tw_r"
  Mux10/1 -> Tw [Nm]/1, Scope3/1
  Saturation1/1 -> Product/2
  Add/1 -> Signed Sqrt/1
  Math Function1/1 -> Add/2

== system FullVehicleModel_ABS_ESP/ABS and Wheel torque generation/Brake ==
  Fpedal [-] : Inport
  Front Brake ratio : Gain  Gain=0.7
  Max Brake Torque : Gain  Gain=1500
  Mux11 : Mux
  Rate Limiter : RateLimiter  RisingSlewLimit=1e5  FallingSlewLimit=-10000  SampleTimeMode=inherited
  Rear Brake ratio : Gain  Gain=0.3
  Saturation : Saturate  UpperLimit=0  LowerLimit=-1
  Tw [Nm] : Outport
  wires:
  Saturation/1 -> Max Brake Torque/1
  Fpedal [-]/1 -> Saturation/1
  Mux11/1 -> Tw [Nm]/1
  Front Brake ratio/1 -> Mux11/4, Mux11/3
  Max Brake Torque/1 -> Rate Limiter/1
  Rate Limiter/1 -> Rear Brake ratio/1, Front Brake ratio/1
  Rear Brake ratio/1 -> Mux11/1, Mux11/2

== system FullVehicleModel_ABS_ESP/Road curvature/Constant curvature Maneuver ==
  Demux : Demux  Tag=STV Demux  Outputs=1
  FromWs : FromWorkspace  Tag=STV FromWs  VariableName=tuvar  SampleTime=0
      SigBuilderData=|
      | common.afterFinalStr = 'Extrapolate'
      | common.sampleTime = 0
      | dataSet.timeRange = [0 20]
      | dataSet.name = 'Group 1'
      | sbobj.Groups.Name = 'Group 1'
      | sbobj.Groups.Signals.Name = 'Signal 1'
      | sbobj.Groups.Signals.XData = [0 0.98 0.98 20]
      | sbobj.Groups.Signals.YData = [0 0 0.4 0.4]
      | sbobj.Groups.TimeRange = [0 20]
  Signal 1 : Outport  Tag=STV Outport
  wires:
  Demux/1 -> Signal 1/1
  FromWs/1 -> Demux/1

== system FullVehicleModel_ABS_ESP/Road curvature/Double Lane Change Maneuver ==
  Demux : Demux  Tag=STV Demux  Outputs=1
  FromWs : FromWorkspace  Tag=STV FromWs  VariableName=tuvar  SampleTime=0
      SigBuilderData=|
      | common.afterFinalStr = 'Extrapolate'
      | common.sampleTime = 0
      | dataSet.timeRange = [0 10]
      | dataSet.name = 'Group 1'
      | sbobj.Groups.Name = 'Group 1'
      | sbobj.Groups.Signals.Name = 'Signal 1'
      | sbobj.Groups.Signals.XData = [0 1 1 1.5 1.5 1.6 1.6 2.1 2.1 3 3 3.5 3.5 3.7 3.7 4.2 4.2 10]
      | sbobj.Groups.Signals.YData = [0 0 0.5 0.5 0 0 -0.504 -0.504 0 0 -0.5 -0.5 0 0 0.5 0.5 0 0]
  Signal 1 : Outport  Tag=STV Outport
  wires:
  FromWs/1 -> Demux/1
  Demux/1 -> Signal 1/1

== system FullVehicleModel_ABS_ESP/Vehicle/Encoders ==
  omega [m/s] : Inport
  Bus Creator : BusCreator  Inputs=4
  Demux : Demux
  Encoders : Outport
  wires:
  omega [m/s]/1 -> Demux/1
  Demux/1 -> Bus Creator/1  "omega_rr"
  Demux/2 -> Bus Creator/2  "omega_rl"
  Demux/3 -> Bus Creator/3  "omega_fr"
  Demux/4 -> Bus Creator/4  "omega_fl"
  Bus Creator/1 -> Encoders/1

== system FullVehicleModel_ABS_ESP/Vehicle/From car2world ref.  ==
  theta : Inport
  u : Inport  Port=2
  v : Inport  Port=3
  Add : Sum  Inputs=+-
  Add1 : Sum
  Product{,1..3} (4 alike) : Product
  Trigonometric Function : Trigonometry  Operator=cos
  Trigonometric Function1 : Trigonometry
  Vx : Outport
  Vy : Outport  Port=2
  wires:
  theta/1 -> Trigonometric Function/1, Trigonometric Function1/1
  u/1 -> Product/1, Product2/1
  Trigonometric Function/1 -> Product3/1, Product/2
  Trigonometric Function1/1 -> Product1/1, Product2/2
  v/1 -> Product3/2, Product1/2
  Product/1 -> Add/1  "u cos(theta)"
  Product1/1 -> Add/2  "v sin(theta)"
  Add/1 -> Vx/1
  Product3/1 -> Add1/1  "v cos(theta)"
  Add1/1 -> Vy/1
  Product2/1 -> Add1/2  "u sin(theta)"

== system FullVehicleModel_ABS_ESP/Vehicle/IMU ==
  u [m/s] : Inport
  v [m/s] : Inport  Port=2
  Omega [rad/s] : Inport  Port=3
  phi_dot [m/s] : Inport  Port=4
  Bus Creator : BusCreator  Inputs=4
  Derivative : Derivative
  Derivative1 : Derivative
  Integrator : Integrator  InitialCondition=V_init/3.6
  Memory : Memory
  Scope : Scope  NumInputPorts=3
  IMU : Outport
  wires:
  u [m/s]/1 -> Derivative/1, Scope/1  "u"
  v [m/s]/1 -> Derivative1/1
  Derivative/1 -> Memory/1  "du_meas"
  Derivative1/1 -> Bus Creator/2  "v_meas"
  Bus Creator/1 -> IMU/1
  Omega [rad/s]/1 -> Bus Creator/3  "Omega"
  phi_dot [m/s]/1 -> Bus Creator/4  "phi_dot"
  Integrator/1 -> Scope/2  "u_int"
  Memory/1 -> Bus Creator/1, Scope/3, Integrator/1

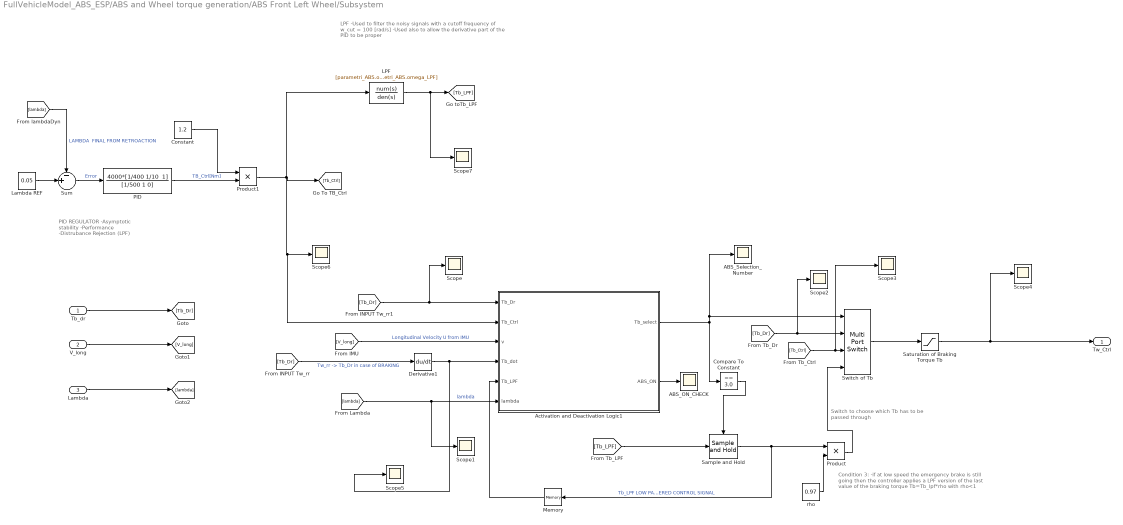
== system FullVehicleModel_ABS_ESP/ABS and Wheel torque generation/ABS Front Left Wheel/Subsystem ==
  note: Condition 3:
      | -if at low speed the emergency brake is still going
      | then the controller applies a LPF version of the last
      | value of the braking torque Tb=Tb_lpf*rho with rho<1
  note: Switch to choose which Tb has to be
      | passed through
  note: LPF
      | -Used to filter the noisy signals with a cutoff frequency of
      | w_cut = 100 [rad/s]
      | -Used also to allow the derivative part of the PID to be proper
  note: PID REGULATOR
      | -Asymptotic stability
      | -Performance
      | -Distrubance Rejection (LPF)
  Tb_dr : Inport
  "V_long " : Inport  Port=2
  Lambda : Inport  Port=3
  ABS_ON_CHECK : Scope
  "ABS_Selection_Number " : Scope
  Activation and Deactivation Logic1 : Stateflow chart  TreatAsAtomicUnit=on
  Compare To Constant : simulink/Logic and Bit Operations/Compare To Constant  relop===  const=3.0  OutDataTypeStr=boolean
  Constant : Constant  Value=1.2
  Derivative1 : Derivative
  LPF : TransferFcn  Numerator=[parametri_ABS.omega_LPF]  Denominator=[1 parametri_ABS.omega_LPF]
  Lambda REF : Constant  Value=0.05
  Memory : Memory
  PID : TransferFcn  Numerator="4000*[1/400 1/10  1]"  Denominator=[1/500 1 0]
  Product : Product
  Product1 : Product
  Sample and Hold : dspsigops/Sample and Hold  trig=Rising edge  initCond=0  latchinput=off
  Saturation of Braking Torque Tb : Saturate  UpperLimit=1500  LowerLimit=0
  Scope{,1..7} (8 alike) : Scope
  Sum : Sum  Inputs=-+|
  Switch of Tb : MultiPortSwitch
  rho : Constant  Value=0.97
  Tw_Ctrl : Outport
  wires:
  Saturation of Braking Torque Tb/1 -> Scope4/1, Tw_Ctrl/1
  rho/1 -> Product/2
  [Tb_Dr] -> Derivative1/1  "Tw_rr -> Tb_Dr in case of BRAKING"
  [Tb_Ctrl] -> Scope3/1, Switch of Tb/3
  Activation and Deactivation Logic1/2(ABS_ON) -> ABS_ON_CHECK/1
  [V_long] -> Activation and Deactivation Logic1/3(v)  "Longitudinal Velocity U from IMU"
  [Tb_Dr] -> Scope2/1, Switch of Tb/2
  Sum/1 -> PID/1  "Error"
  Compare To Constant/1 -> Sample and Hold/Trigger
  Derivative1/1 -> Scope5/1, Activation and Deactivation Logic1/4(Tb_dot)
  [Tb_LPF] -> Sample and Hold/1
  Sample and Hold/1 -> Memory/1, Product/1  "Tb_LPF LOW PASS  FILTERED CONTROL SIGNAL"
  [Tb_Dr] -> Scope/1, Activation and Deactivation Logic1/1(Tb_Dr)
  Activation and Deactivation Logic1/1(Tb_select) -> Compare To Constant/1, Switch of Tb/1, "ABS_Selection_Number "/1
  Product/1 -> Switch of Tb/4
  Switch of Tb/1 -> Saturation of Braking Torque Tb/1
  Memory/1 -> Activation and Deactivation Logic1/5(Tb_LPF)
  LPF/1 -> Scope7/1, [Tb_LPF]
  Tb_dr/1 -> [Tb_Dr]
  "V_long "/1 -> [V_long]
  Lambda/1 -> [lambda]
  Lambda REF/1 -> Sum/2
  [lambda] -> Sum/1  "LAMBDA  FINAL FROM RETROACTION"
  [lambda] -> Scope1/1, Activation and Deactivation Logic1/6(lambda)  "lambda"
  PID/1 -> Product1/2  "TB_Ctrl[Nm]"
  Constant/1 -> Product1/1
  Product1/1 -> Activation and Deactivation Logic1/2(Tb_Ctrl), Scope6/1, LPF/1, [Tb_Ctrl]

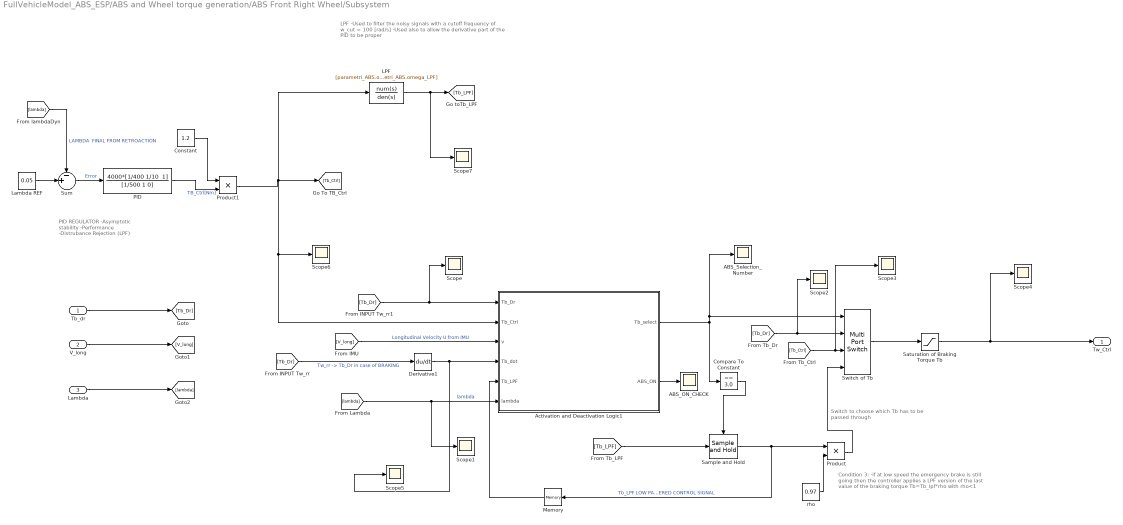
== system FullVehicleModel_ABS_ESP/ABS and Wheel torque generation/ABS Front Right Wheel/Subsystem ==
  note: Condition 3:
      | -if at low speed the emergency brake is still going
      | then the controller applies a LPF version of the last
      | value of the braking torque Tb=Tb_lpf*rho with rho<1
  note: Switch to choose which Tb has to be
      | passed through
  note: LPF
      | -Used to filter the noisy signals with a cutoff frequency of
      | w_cut = 100 [rad/s]
      | -Used also to allow the derivative part of the PID to be proper
  note: PID REGULATOR
      | -Asymptotic stability
      | -Performance
      | -Distrubance Rejection (LPF)
  Tb_dr : Inport
  "V_long " : Inport  Port=2
  Lambda : Inport  Port=3
  ABS_ON_CHECK : Scope
  "ABS_Selection_Number " : Scope
  Activation and Deactivation Logic1 : Stateflow chart  TreatAsAtomicUnit=on
  Compare To Constant : simulink/Logic and Bit Operations/Compare To Constant  relop===  const=3.0  OutDataTypeStr=boolean
  Constant : Constant  Value=1.2
  Derivative1 : Derivative
  LPF : TransferFcn  Numerator=[parametri_ABS.omega_LPF]  Denominator=[1 parametri_ABS.omega_LPF]
  Lambda REF : Constant  Value=0.05
  Memory : Memory
  PID : TransferFcn  Numerator="4000*[1/400 1/10  1]"  Denominator=[1/500 1 0]
  Product : Product
  Product1 : Product
  Sample and Hold : dspsigops/Sample and Hold  trig=Rising edge  initCond=0  latchinput=off
  Saturation of Braking Torque Tb : Saturate  UpperLimit=1500  LowerLimit=0
  Scope{,1..7} (8 alike) : Scope
  Sum : Sum  Inputs=-+|
  Switch of Tb : MultiPortSwitch
  rho : Constant  Value=0.97
  Tw_Ctrl : Outport
  wires:
  Saturation of Braking Torque Tb/1 -> Scope4/1, Tw_Ctrl/1
  rho/1 -> Product/2
  [Tb_Dr] -> Derivative1/1  "Tw_rr -> Tb_Dr in case of BRAKING"
  [Tb_Ctrl] -> Scope3/1, Switch of Tb/3
  Activation and Deactivation Logic1/2(ABS_ON) -> ABS_ON_CHECK/1
  [V_long] -> Activation and Deactivation Logic1/3(v)  "Longitudinal Velocity U from IMU"
  [Tb_Dr] -> Scope2/1, Switch of Tb/2
  Sum/1 -> PID/1  "Error"
  Compare To Constant/1 -> Sample and Hold/Trigger
  Derivative1/1 -> Scope5/1, Activation and Deactivation Logic1/4(Tb_dot)
  [Tb_LPF] -> Sample and Hold/1
  Sample and Hold/1 -> Memory/1, Product/1  "Tb_LPF LOW PASS  FILTERED CONTROL SIGNAL"
  [Tb_Dr] -> Scope/1, Activation and Deactivation Logic1/1(Tb_Dr)
  Activation and Deactivation Logic1/1(Tb_select) -> Compare To Constant/1, Switch of Tb/1, "ABS_Selection_Number "/1
  Product/1 -> Switch of Tb/4
  Switch of Tb/1 -> Saturation of Braking Torque Tb/1
  Memory/1 -> Activation and Deactivation Logic1/5(Tb_LPF)
  LPF/1 -> Scope7/1, [Tb_LPF]
  Tb_dr/1 -> [Tb_Dr]
  "V_long "/1 -> [V_long]
  Lambda/1 -> [lambda]
  Lambda REF/1 -> Sum/2
  [lambda] -> Sum/1  "LAMBDA  FINAL FROM RETROACTION"
  [lambda] -> Scope1/1, Activation and Deactivation Logic1/6(lambda)  "lambda"
  Constant/1 -> Product1/1
  PID/1 -> Product1/2  "TB_Ctrl[Nm]"
  Product1/1 -> Activation and Deactivation Logic1/2(Tb_Ctrl), Scope6/1, LPF/1, [Tb_Ctrl]

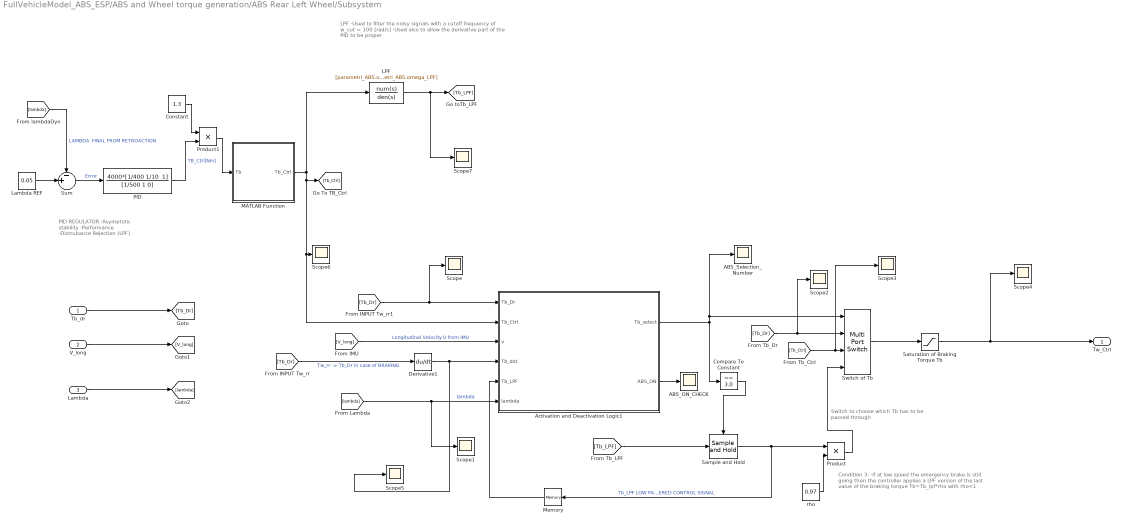
== system FullVehicleModel_ABS_ESP/ABS and Wheel torque generation/ABS Rear Left Wheel/Subsystem ==
  note: Condition 3:
      | -if at low speed the emergency brake is still going
      | then the controller applies a LPF version of the last
      | value of the braking torque Tb=Tb_lpf*rho with rho<1
  note: Switch to choose which Tb has to be
      | passed through
  note: LPF
      | -Used to filter the noisy signals with a cutoff frequency of
      | w_cut = 100 [rad/s]
      | -Used also to allow the derivative part of the PID to be proper
  note: PID REGULATOR
      | -Asymptotic stability
      | -Performance
      | -Distrubance Rejection (LPF)
  Tb_dr : Inport
  "V_long " : Inport  Port=2
  Lambda : Inport  Port=3
  ABS_ON_CHECK : Scope
  "ABS_Selection_Number " : Scope
  Activation and Deactivation Logic1 : Stateflow chart  TreatAsAtomicUnit=on
  Compare To Constant : simulink/Logic and Bit Operations/Compare To Constant  relop===  const=3.0  OutDataTypeStr=boolean
  Constant : Constant  Value=1.3
  Derivative1 : Derivative
  LPF : TransferFcn  Numerator=[parametri_ABS.omega_LPF]  Denominator=[1 parametri_ABS.omega_LPF]
  Lambda REF : Constant  Value=0.05
  MATLAB Function : MATLAB Function  TreatAsAtomicUnit=on
  Memory : Memory
  PID : TransferFcn  Numerator="4000*[1/400 1/10  1]"  Denominator=[1/500 1 0]
  Product : Product
  Product1 : Product
  Sample and Hold : dspsigops/Sample and Hold  trig=Rising edge  initCond=0  latchinput=off
  Saturation of Braking Torque Tb : Saturate  UpperLimit=1500  LowerLimit=-10000
  Scope{,1..7} (8 alike) : Scope
  Sum : Sum  Inputs=-+|
  Switch of Tb : MultiPortSwitch
  rho : Constant  Value=0.97
  Tw_Ctrl : Outport
  wires:
  Saturation of Braking Torque Tb/1 -> Scope4/1, Tw_Ctrl/1
  rho/1 -> Product/2
  [Tb_Dr] -> Derivative1/1  "Tw_rr -> Tb_Dr in case of BRAKING"
  [Tb_Ctrl] -> Scope3/1, Switch of Tb/3
  Activation and Deactivation Logic1/2(ABS_ON) -> ABS_ON_CHECK/1
  [V_long] -> Activation and Deactivation Logic1/3(v)  "Longitudinal Velocity U from IMU"
  [Tb_Dr] -> Scope2/1, Switch of Tb/2
  Sum/1 -> PID/1  "Error"
  Compare To Constant/1 -> Sample and Hold/Trigger
  Derivative1/1 -> Scope5/1, Activation and Deactivation Logic1/4(Tb_dot)
  [Tb_LPF] -> Sample and Hold/1
  Sample and Hold/1 -> Memory/1, Product/1  "Tb_LPF LOW PASS  FILTERED CONTROL SIGNAL"
  [Tb_Dr] -> Scope/1, Activation and Deactivation Logic1/1(Tb_Dr)
  Activation and Deactivation Logic1/1(Tb_select) -> Compare To Constant/1, Switch of Tb/1, "ABS_Selection_Number "/1
  Product/1 -> Switch of Tb/4
  Switch of Tb/1 -> Saturation of Braking Torque Tb/1
  Memory/1 -> Activation and Deactivation Logic1/5(Tb_LPF)
  LPF/1 -> Scope7/1, [Tb_LPF]
  Tb_dr/1 -> [Tb_Dr]
  "V_long "/1 -> [V_long]
  Lambda/1 -> [lambda]
  Lambda REF/1 -> Sum/2
  [lambda] -> Sum/1  "LAMBDA  FINAL FROM RETROACTION"
  [lambda] -> Scope1/1, Activation and Deactivation Logic1/6(lambda)  "lambda"
  MATLAB Function/1(Tb_Ctrl) -> Activation and Deactivation Logic1/2(Tb_Ctrl), Scope6/1, [Tb_Ctrl], LPF/1
  Constant/1 -> Product1/1
  PID/1 -> Product1/2  "TB_Ctrl[Nm]"
  Product1/1 -> MATLAB Function/1(Tb)

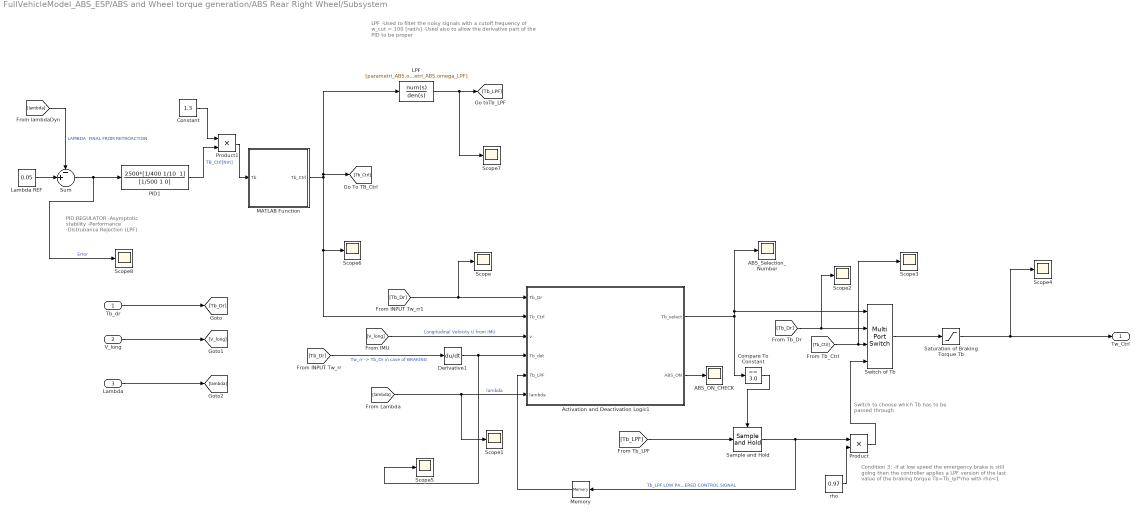
== system FullVehicleModel_ABS_ESP/ABS and Wheel torque generation/ABS Rear Right Wheel/Subsystem ==
  note: Condition 3:
      | -if at low speed the emergency brake is still going
      | then the controller applies a LPF version of the last
      | value of the braking torque Tb=Tb_lpf*rho with rho<1
  note: Switch to choose which Tb has to be
      | passed through
  note: LPF
      | -Used to filter the noisy signals with a cutoff frequency of
      | w_cut = 100 [rad/s]
      | -Used also to allow the derivative part of the PID to be proper
  note: PID REGULATOR
      | -Asymptotic stability
      | -Performance
      | -Distrubance Rejection (LPF)
  Tb_dr : Inport
  "V_long " : Inport  Port=2
  Lambda : Inport  Port=3
  ABS_ON_CHECK : Scope
  "ABS_Selection_Number " : Scope
  Activation and Deactivation Logic1 : Stateflow chart  TreatAsAtomicUnit=on
  Compare To Constant : simulink/Logic and Bit Operations/Compare To Constant  relop===  const=3.0  OutDataTypeStr=boolean
  Constant : Constant  Value=1.3
  Derivative1 : Derivative
  LPF : TransferFcn  Numerator=[parametri_ABS.omega_LPF]  Denominator=[1 parametri_ABS.omega_LPF]
  Lambda REF : Constant  Value=0.05
  MATLAB Function : MATLAB Function  TreatAsAtomicUnit=on
  Memory : Memory
  PID1 : TransferFcn  Numerator="2500*[1/400 1/10  1]"  Denominator=[1/500 1 0]
  Product : Product
  Product1 : Product
  Sample and Hold : dspsigops/Sample and Hold  trig=Rising edge  initCond=0  latchinput=off
  Saturation of Braking Torque Tb : Saturate  UpperLimit=1500  LowerLimit=-10000
  Scope{,1..8} (9 alike) : Scope
  Sum : Sum  Inputs=-+|
  Switch of Tb : MultiPortSwitch
  rho : Constant  Value=0.97
  Tw_Ctrl : Outport
  wires:
  Saturation of Braking Torque Tb/1 -> Scope4/1, Tw_Ctrl/1
  rho/1 -> Product/2
  [Tb_Dr] -> Derivative1/1  "Tw_rr -> Tb_Dr in case of BRAKING"
  [Tb_Ctrl] -> Scope3/1, Switch of Tb/3
  Activation and Deactivation Logic1/2(ABS_ON) -> ABS_ON_CHECK/1
  [V_long] -> Activation and Deactivation Logic1/3(v)  "Longitudinal Velocity U from IMU"
  [Tb_Dr] -> Scope2/1, Switch of Tb/2
  Sum/1 -> Scope8/1, PID1/1  "Error"
  Compare To Constant/1 -> Sample and Hold/Trigger
  Derivative1/1 -> Scope5/1, Activation and Deactivation Logic1/4(Tb_dot)
  [Tb_LPF] -> Sample and Hold/1
  Sample and Hold/1 -> Memory/1, Product/1  "Tb_LPF LOW PASS  FILTERED CONTROL SIGNAL"
  [Tb_Dr] -> Scope/1, Activation and Deactivation Logic1/1(Tb_Dr)
  Activation and Deactivation Logic1/1(Tb_select) -> Compare To Constant/1, Switch of Tb/1, "ABS_Selection_Number "/1
  Product/1 -> Switch of Tb/4
  Switch of Tb/1 -> Saturation of Braking Torque Tb/1
  Memory/1 -> Activation and Deactivation Logic1/5(Tb_LPF)
  LPF/1 -> Scope7/1, [Tb_LPF]
  Tb_dr/1 -> [Tb_Dr]
  "V_long "/1 -> [V_long]
  Lambda/1 -> [lambda]
  Lambda REF/1 -> Sum/2
  [lambda] -> Sum/1  "LAMBDA  FINAL FROM RETROACTION"
  [lambda] -> Scope1/1, Activation and Deactivation Logic1/6(lambda)  "lambda"
  MATLAB Function/1(Tb_Ctrl) -> Activation and Deactivation Logic1/2(Tb_Ctrl), Scope6/1, LPF/1, [Tb_Ctrl]
  PID1/1 -> Product1/2  "TB_Ctrl[Nm]"
  Constant/1 -> Product1/1
  Product1/1 -> MATLAB Function/1(Tb)

== matlab function FullVehicleModel_ABS_ESP/ABS and Wheel torque generation/ABS Rear Left Wheel/MATLAB Function ==
  data: lambda input; RHS output; Tb input; v input; vehicle_data parameter; Fz input
function RHS = lambdaDyn(lambda,Tb,v,vehicle_data,Fz)

omega = (1-lambda)*v/vehicle_data.rear_wheel.Rr;

%Psi = (vehicle_data.rear_wheel.Rr+vehicle_data.rear_wheel.iwd_r/(vehicle_data.rear_wheel.iwd_r*vehicle_data.vehicle.m)*(1-lambda))*Fz*1.2*burckhardt(lambda,1);
Psi=vehicle_data.rear_wheel.Rr*Fz*burckhardt(lambda,1);

if omega<=1
    RHS=0;
else
    RHS=-((1-lambda)/(vehicle_data.rear_wheel.iwd_r*omega))*(Psi-Tb);
end

end

== matlab function FullVehicleModel_ABS_ESP/ABS and Wheel torque generation/ABS Rear Right Wheel/MATLAB Function ==
  data: lambda input; RHS output; Tb input; v input; vehicle_data parameter; Fz input; Psi output
function [RHS,Psi]= lambdaDyn(lambda,Tb,v,vehicle_data,Fz)

omega = (1-lambda)*v/vehicle_data.rear_wheel.Rr;

%Psi = (vehicle_data.rear_wheel.Rr+vehicle_data.rear_wheel.iwd_r/(vehicle_data.rear_wheel.iwd_r*vehicle_data.vehicle.m)*(1-lambda))*Fz*1.258*burckhardt(lambda,1);
Psi=vehicle_data.rear_wheel.Rr*Fz*burckhardt(lambda,1);

if omega<=1
    RHS=0;
else
    RHS=-((1-lambda)/(vehicle_data.rear_wheel.iwd_r*omega))*(Psi-Tb);
end

end

== stateflow chart FullVehicleModel_ABS_ESP/ABS and Wheel torque generation/ABS Rear Left Wheel/Subsystem/Activation and Deactivation Logic1 ==
  state High_Speed_ON
    entry: Tb_select = 2;
    entry: ABS_ON = true;
  state High_Speed_OFF
    entry: Tb_select = 1;
    entry: ABS_ON = false;
  state Low_Speed_ON
    entry: Tb_select = 3;
    entry: ABS_ON = true;
  state Low_Speed_OFF
    entry: Tb_select = 1;
    entry: ABS_ON = false;
  High_Speed_OFF -> High_Speed_ON [order 1] : [lambda > lambda1_th - ((lambda1_th - lambda2_th)/1500)*Tb_dot && ...
      |  Tb_Dr > rho_on*Tb_Ctrl && ...
      |  v > v_on]
  (default) -> High_Speed_OFF : {Tb_select = 1;}
  High_Speed_ON -> High_Speed_OFF [order 1] : [Tb_Dr < rho_off*Tb_Ctrl]
  High_Speed_OFF -> Low_Speed_OFF [order 2] : [v < v_on -hv]
  Low_Speed_OFF -> High_Speed_OFF : [v > v_on +hv]
  High_Speed_ON -> Low_Speed_ON [order 2] : [v < v_on]
  Low_Speed_ON -> Low_Speed_OFF : [v < v_stop || Tb_Dr < rho_off*Tb_LPF]
  data: Tb_select output; Tb_Dr input; Tb_Ctrl input; v input; Tb_dot input; Tb_dot_max parameter; v_on parameter; rho_on parameter; Tb_LPF input; lambda input; lambda1_th parameter; v_stop parameter; hv parameter; rho_off parameter; ABS_ON output; lambda2_th parameter

== matlab function FullVehicleModel_ABS_ESP/ABS and Wheel torque generation/ABS Front Right Wheel/MATLAB Function ==
  data: lambda input; RHS output; Tb input; v input; vehicle_data parameter; Fz input
function RHS = lambdaDyn(lambda,Tb,v,vehicle_data,Fz)

omega = (1-lambda)*v/vehicle_data.front_wheel.Rf;

Psi = (vehicle_data.front_wheel.Rf+vehicle_data.front_wheel.iwd_f/(vehicle_data.front_wheel.iwd_f*vehicle_data.vehicle.m)*(1-lambda))*Fz*1.5*burckhardt(lambda,1);

if omega<=1
    RHS=0;
else
    RHS=-((1-lambda)/(vehicle_data.front_wheel.iwd_f*omega))*(Psi-Tb);
end

end

== stateflow chart FullVehicleModel_ABS_ESP/ABS and Wheel torque generation/ABS Front Right Wheel/Subsystem/Activation and Deactivation Logic1 ==
  state High_Speed_ON
    entry: Tb_select = 2;
    entry: ABS_ON = true;
  state High_Speed_OFF
    entry: Tb_select = 1;
    entry: ABS_ON = false;
  state Low_Speed_ON
    entry: Tb_select = 3;
    entry: ABS_ON = true;
  state Low_Speed_OFF
    entry: Tb_select = 1;
    entry: ABS_ON = false;
  High_Speed_OFF -> High_Speed_ON [order 1] : [lambda > lambda1_th - ((lambda1_th - lambda2_th)/3000)*Tb_dot && ...
      |  Tb_Dr > rho_on*Tb_Ctrl && ...
      |  v > v_on]
  (default) -> High_Speed_OFF : {Tb_select = 1;}
  High_Speed_ON -> High_Speed_OFF [order 1] : [Tb_Dr < rho_off*Tb_Ctrl]
  High_Speed_OFF -> Low_Speed_OFF [order 2] : [v < v_on -hv]
  Low_Speed_OFF -> High_Speed_OFF : [v > v_on +hv]
  High_Speed_ON -> Low_Speed_ON [order 2] : [v < v_on]
  Low_Speed_ON -> Low_Speed_OFF : [v < v_stop || Tb_Dr < rho_off*Tb_LPF]
  data: Tb_select output; Tb_Dr input; Tb_Ctrl input; v input; Tb_dot input; Tb_dot_max parameter; v_on parameter; rho_on parameter; Tb_LPF input; lambda input; lambda1_th parameter; v_stop parameter; hv parameter; rho_off parameter; ABS_ON output; lambda2_th parameter
